simulink model "ClosedLoopAngular"  (R2019a)
settings: Solver=VariableStepAuto  StartTime=0.0  StopTime=50.0  RelTol=1e-3
values from neighbouring files (symbols this model uses):
  den1 = [taum 1]    [classical.m]
  Kdin = (2*zetacin*wcin*Tm-1)/Km    [classical.m]
  Kpin = wcin^2*Tm/(Kdin*Km)    [classical.m]
  num1 = [Km1]    [classical.m]
  wanttheta1 = 10    [classical.m]
  wanttheta2 = 30    [classical.m]
settings Model: Creator=xde12  LastModifiedBy=xde12

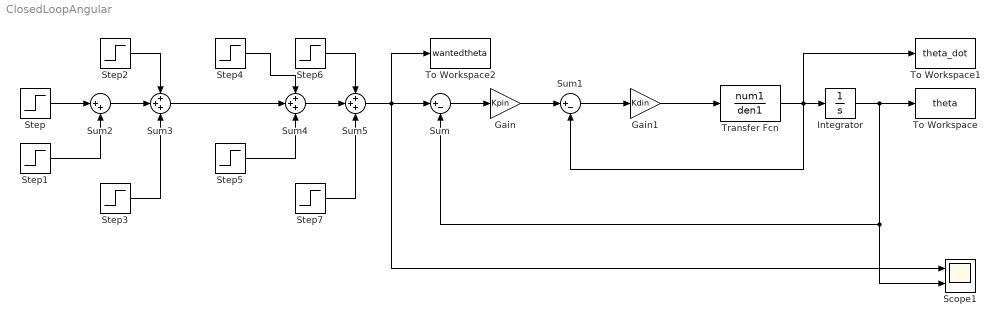
== system ClosedLoopAngular ==
  Gain : Gain  Gain=Kpin
  Gain1 : Gain  Gain=Kdin
  Integrator : Integrator
  Scope1 : Scope  NumInputPorts=2
  Step : Step  Time=5  After=wanttheta1  SampleTime=0
  Step1 : Step  Time=10  After=-wanttheta1  SampleTime=0
  Step2 : Step  Time=15  After=-wanttheta1  SampleTime=0
  Step3 : Step  Time=20  After=wanttheta1  SampleTime=0
  Step4 : Step  Time=25  After=wanttheta2  SampleTime=0
  Step5 : Step  Time=30  After=-wanttheta2  SampleTime=0
  Step6 : Step  Time=35  After=-wanttheta2  SampleTime=0
  Step7 : Step  Time=40  After=wanttheta2  SampleTime=0
  Sum : Sum  Inputs=|+-
  Sum1 : Sum  Inputs=|+-
  Sum2 : Sum  Inputs=|++
  Sum3 : Sum  Inputs=+++
  Sum4 : Sum  Inputs=+++
  Sum5 : Sum  Inputs=+++
  To Workspace : ToWorkspace  VariableName=theta  SampleTime=-1
  To Workspace1 : ToWorkspace  VariableName=theta_dot  SampleTime=-1
  To Workspace2 : ToWorkspace  VariableName=wantedtheta  SampleTime=-1
  Transfer Fcn : TransferFcn  Numerator=num1  Denominator=den1
  wires:
  Gain/1 -> Sum1/1
  Sum1/1 -> Gain1/1
  Gain1/1 -> Transfer Fcn/1
  Transfer Fcn/1 -> To Workspace1/1, Sum1/2, Integrator/1
  Integrator/1 -> To Workspace/1, Scope1/2, Sum/2
  Sum/1 -> Gain/1
  Step/1 -> Sum2/1
  Step1/1 -> Sum2/2
  Sum2/1 -> Sum3/2
  Step2/1 -> Sum3/1
  Step3/1 -> Sum3/3
  Step6/1 -> Sum5/1
  Step7/1 -> Sum5/3
  Sum4/1 -> Sum5/2
  Step4/1 -> Sum4/1
  Step5/1 -> Sum4/3
  Sum3/1 -> Sum4/2
  Sum5/1 -> To Workspace2/1, Scope1/1, Sum/1
